simulink model "DCMotor_sim"  (R2019a)
settings: Solver=VariableStepAuto  StartTime=0.0  StopTime=simEnd  FixedStep=T  MaxStep=T  RelTol=1e-3
values from neighbouring files (symbols this model uses):
  A = [-Ra/La -Kt/La ... (first row only)    [getMotorStateSpace.m]
  B = [1/La 0 ... (first row only)    [getMotorStateSpace.m]
  C = [1 0 ... (first row only)    [getMotorStateSpace.m]    (also in getPIDValues.m = pidtune(system, 'PID'))
  D = [0 0 ... (first row only)    [getMotorStateSpace.m]
  T = 0.001    [DCMotorFault.m]    (also in GenerateMotorFault.m; GenerateMotorValues.m; SetupMotor.m)
settings Model: Creator=alexc  LastModifiedBy=alexc

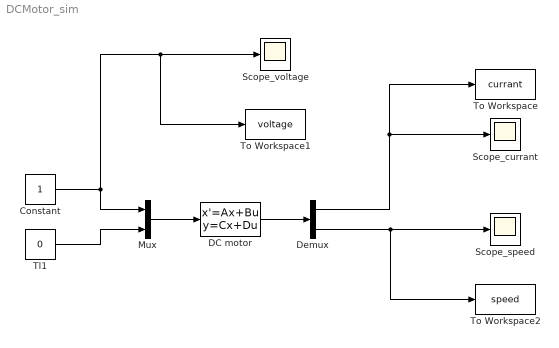
== system DCMotor_sim ==
  Constant : Constant
  DC motor : StateSpace  A=A  B=B  C=C  D=D  InitialCondition=0
  Demux : Demux  Outputs=2
  Mux : Mux  Inputs=2
  Scope_currant : Scope
  Scope_speed : Scope
  Scope_voltage : Scope
  Tl1 : Constant  Value=0
  To Workspace : ToWorkspace  VariableName=currant  SaveFormat=Timeseries  SampleTime=T
  To Workspace1 : ToWorkspace  VariableName=voltage  SaveFormat=Timeseries  SampleTime=T
  To Workspace2 : ToWorkspace  VariableName=speed  SaveFormat=Timeseries  SampleTime=T
  wires:
  Demux/2 -> Scope_speed/1, To Workspace2/1
  Demux/1 -> To Workspace/1, Scope_currant/1
  Tl1/1 -> Mux/2
  DC motor/1 -> Demux/1
  Mux/1 -> DC motor/1
  Constant/1 -> Mux/1, Scope_voltage/1, To Workspace1/1
